simulink model "Smart_City_QCar2_self_driving_stack"  (R2024b)
settings: Solver=ode1  StartTime=0.0  StopTime=inf  FixedStep=Controller_Sample_Time  RelTol=1e-3  EnableMultiTasking=on
values from neighbouring files (symbols this model uses):
  angles_qcar2 = angles_new_qcar2(2: length (angles_new_qcar2), width (angles_new_qcar2)-5)    [Setup_QCar1and2_params.m]
  Audio_Sample_Time = 0.3    [Setup_QCar1and2_params.m]
  cal_pos = [0, 0, 0]    [Setup_QCar1and2_params.m]
  cameraStepSize = 3e-2    (= 0.03)    [Setup_QCar1and2_params.m]
  Cobra_Start = [0 0 0 0 0 0 0 0 0 0 0 0 ... (192000 elements, 192000x1)]    [QCar_Sounds.mat]
  Controller_Sample_Time = CSI_Sample_Time/10    (= 0.00166666666667)    [Setup_QCar1and2_params.m]
  CSI_Sample_Time = 1/60    (= 0.0166666666667)    [Setup_QCar1and2_params.m]
  engine = [0.455749511719 0.619506835938 0.612854003906 0.499603271484 0.347473144531 0.278045654297 0.304656982422 0.258544921875 0.100128173828 0.0902099609375 0.341461181641 0.515716552734 ... (88200 elements, 44100x2)]    [QCar_Sounds.mat]
  GyroKF_P0 = eye(2)    [Setup_QCar1and2_params.m]
  GyroKF_Q = diag([0.01, 0.001])    [Setup_QCar1and2_params.m]
  GyroKF_R = 0.01    [Setup_QCar1and2_params.m]
  GyroKF_X0 = [0;0]    [Setup_QCar1and2_params.m]
  honk = [0.01708984375 0.0179443359375 0.018798828125 0.019775390625 0.0209655761719 0.0218505859375 0.0221557617188 0.0223693847656 0.022705078125 0.023681640625 0.0252075195312 0.0257263183594 ... (43568 elements, 21784x2)]    [QCar_Sounds.mat]
  ImageDisplay_Sample_Time = CSI_Sample_Time*6    (= 0.1)    [Setup_QCar1and2_params.m]
  Initialization_Time = 5    [Setup_QCar1and2_params.m]
  LiDAR_Sample_Time = CSI_Sample_Time*3    (= 0.05)    [Setup_QCar1and2_params.m]
  map_mask = [1 1 1 0 0 1 0]    [Setup_QCar1and2_params.m]
  NN_Sample_Time = RealSense_Sample_Time*1    (= 0.0333333333333)    [Setup_QCar1and2_params.m]
  path_x = [0.826 0.836 0.846 0.856 0.866 0.876 0.886 0.896 0.906 0.916 0.926 0.936 ... (740 elements, 740x1)]    [SDCS_Paths_7.mat]
  path_x2 = [-0.614 -0.604 -0.594 -0.584 -0.574 -0.564 -0.554 -0.544 -0.534 -0.524 -0.514 -0.504 ... (1090 elements, 1090x1)]    [SDCS_Paths_7.mat]
  path_x3 = [-0.614 -0.603821428571 -0.593642857143 -0.583464285714 -0.573285714286 -0.563107142857 -0.552928571429 -0.54275 -0.532571428571 -0.522392857143 -0.512214285714 -0.502035714286 ... (714 elements, 714x1)]    [SDCS_Paths_7.mat]
  path_x4 = [-0.614 -0.604 -0.594 -0.584 -0.574 -0.564 -0.554 -0.544 -0.534 -0.524 -0.514 -0.504 ... (1761 elements, 1761x1)]    [SDCS_Paths_7.mat]
  path_x5 = [1.436 1.42588571429 1.41577142857 1.40565714286 1.39554285714 1.38542857143 1.37531428571 1.3652 1.35508571429 1.34497142857 1.33485714286 1.32474285714 ... (574 elements, 574x1)]    [SDCS_Paths_7.mat]
  path_x6 = [1.436 1.42588571429 1.41577142857 1.40565714286 1.39554285714 1.38542857143 1.37531428571 1.3652 1.35508571429 1.34497142857 1.33485714286 1.32474285714 ... (1288 elements, 1288x1)]    [SDCS_Paths_7.mat]
  path_x7 = [-1.5778487585 -1.56959877056 -1.56127865467 -1.55288878259 -1.54442952915 -1.53590127231 -1.52730439309 -1.51863927561 -1.50990630701 -1.50110587746 -1.49223838016 -1.4833042113 ... (2260 elements, 2260x1)]    [SDCS_Paths_7.mat]
  path_y = [-1.0887 -1.0887 -1.0887 -1.0887 -1.0887 -1.0887 -1.0887 -1.0887 -1.0887 -1.0887 -1.0887 -1.0887 ... (740 elements, 740x1)]    [SDCS_Paths_7.mat]
  path_y2 = [-1.0887 -1.0887 -1.0887 -1.0887 -1.0887 -1.0887 -1.0887 -1.0887 -1.0887 -1.0887 -1.0887 -1.0887 ... (1090 elements, 1090x1)]    [SDCS_Paths_7.mat]
  path_y3 = [-1.0887 -1.0887 -1.0887 -1.0887 -1.0887 -1.0887 -1.0887 -1.0887 -1.0887 -1.0887 -1.0887 -1.0887 ... (714 elements, 714x1)]    [SDCS_Paths_7.mat]
  path_y4 = [-1.0887 -1.0887 -1.0887 -1.0887 -1.0887 -1.0887 -1.0887 -1.0887 -1.0887 -1.0887 -1.0887 -1.0887 ... (1761 elements, 1761x1)]    [SDCS_Paths_7.mat]
  path_y5 = [-0.8157 -0.8157 -0.8157 -0.8157 -0.8157 -0.8157 -0.8157 -0.8157 -0.8157 -0.8157 -0.8157 -0.8157 ... (574 elements, 574x1)]    [SDCS_Paths_7.mat]
  path_y6 = [-0.8157 -0.8157 -0.8157 -0.8157 -0.8157 -0.8157 -0.8157 -0.8157 -0.8157 -0.8157 -0.8157 -0.8157 ... (1288 elements, 1288x1)]    [SDCS_Paths_7.mat]
  path_y7 = [-0.614490295955 -0.61974988896 -0.624981792226 -0.630185771997 -0.635361595765 -0.640509032279 -0.645627851559 -0.6507178249 -0.655778724888 -0.660810325409 -0.665812401655 -0.670784730139 ... (2260 elements, 2260x1)]    [SDCS_Paths_7.mat]
  put_me_down = [0 0 0 0 0 0 0 0 0 0 0 0 ... (335870 elements, 167935x2)]    [QCar_Sounds.mat]
  qcar2_lidar_to_map_rotation = 0    [Setup_QCar1and2_params.m]
  QCarEKF_L = 0.24    [Setup_QCar1and2_params.m]
  QCarEKF_P0 = eye(3)    [Setup_QCar1and2_params.m]
  QCarEKF_Q = diag([0.00001, 0.00001, 0.00001])    [Setup_QCar1and2_params.m]
  QCarEKF_R_combined = diag([0.1, 0.1, 0.01])    [Setup_QCar1and2_params.m]
  QCarEKF_R_heading = diag(0.1)    [Setup_QCar1and2_params.m]
  QcarKF_X0 = [0; 0; 0]    [Setup_QCar1and2_params.m]
  range_qcar2 = distance_new_qcar2(2: length (distance_new_qcar2), width (distance_new_qcar2)-5)    [Setup_QCar1and2_params.m]
  RealSense_Sample_Time = CSI_Sample_Time*2    (= 0.0333333333333)    [Setup_QCar1and2_params.m]
  truck_start = [0.00137329101562 0.00115966796875 0.0006103515625 0.000762939453125 0.00115966796875 0.00198364257812 0.00115966796875 0.000762939453125 0.00137329101562 0.00115966796875 0.00115966796875 0.000762939453125 ... (60000 elements, 60000x1)]    [QCar_Sounds.mat]
undefined symbols (not defined in the file or in its folder): DiscIntNeverNeededParam, gcbh, height, HIL, Joystick_Sample_Time, JPEG, left, Point, qc_get_step_size, top, video_display_show, width
libraries: quarc_library x65, simulink_extras x12, simulink x8
(part 1 of 5)
settings Model: SimulationMode=external  ExtModeTrigDuration=10000  Creator=PKaram  LastModifiedBy=user
settings SolverCC: AlgebraicLoopSolver=TrustRegion  PositivePriorityOrder=on  AutoInsertRateTranBlk=on
settings DataIOCC: ReturnWorkspaceOutputs=off
settings DebuggingCC: ParameterPrecisionLossMsg=none  UnconnectedInputMsg=warning  UnconnectedOutputMsg=warning  UnconnectedLineMsg=warning  ArithmeticOperatorsInVariantConditions=warning
settings HardwareCC: ProdBitPerLong=64  ProdLargestAtomicInteger=LongLong  ProdLargestAtomicFloat=Double  ProdLongLongMode=on  ProdHWDeviceType=ARM Compatible->ARM 64-bit (LP64)
settings ModelReferenceCC: EnableRefExpFcnMdlSchedulingChecks=on
settings SFSimCC: SimUseLocalCustomCode=off  CustomCodeUndefinedFunction=UseInterfaceOnly
settings RTWCC: Description=QUARC Linux QCar2 Target Using Toolchain  SystemTargetFile=quarc_linux_qcar2.tlc  TemplateMakefile=quarc_linux_nvidia_tmf  RTWUseLocalCustomCode=off  Toolchain=QUARC linux_qcar2 | gmake (64-bit Windows)  BuildConfiguration=Faster Runs  GPUComputeCapability=3.5  DLArmComputeVersion=19.05
settings CodeAppCC: StateflowObjectComments=on
settings STFCustomTargetCC: TargetLangStandard=C99 (ISO)  ConcurrentExecutionCompliant=on  GRTInterface=on  UseToolchainInfoCompliant=on  SystemTargetFile=quarc_linux_qcar2.tlc
settings GRTTargetCC: ParMdlRefBuildCompliant=off  CompOptLevelCompliant=off  CombineOutputUpdateFcns=off  MatFileLogging=off  CPPClassGenCompliant=off  GRTInterface=on  ExtMode=on  ExtModeMexFile=quarc_comm  ExtModeMexArgs='-w -d /home/nvidia/Documents -uri %u', 'tcpip://192.168.2.11:17001'
settings ConfigComp: CovMetricSettings=dswe

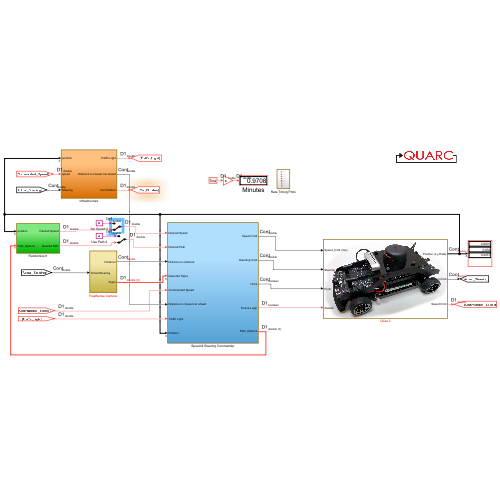
[thumbnail: Simulink's stored preview of the top-level diagram]
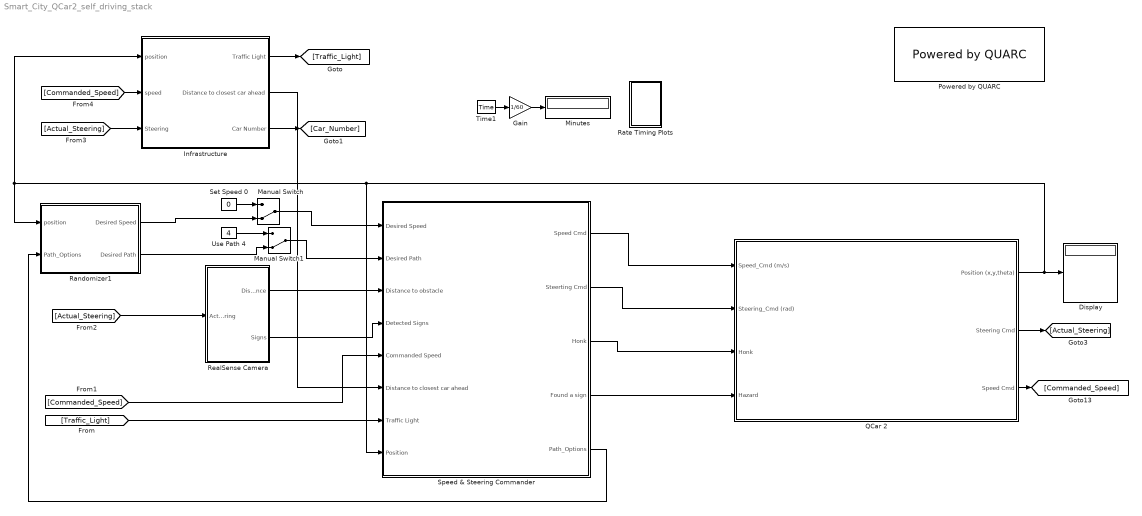
== system Smart_City_QCar2_self_driving_stack ==
  Display : Display
  Gain : Gain  Gain=1/60
  Infrastructure : Subsystem
  Manual Switch : ManualSwitch  CurrentSetting=0
  Manual Switch1 : ManualSwitch  CurrentSetting=0
  Minutes : Display
  Powered by QUARC : quarc_library/Logos/Powered by QUARC
  QCar 2 : Subsystem
      mask Display: image('QCar2.png');
  Randomizer1 : Subsystem
  Rate Timing Plots : Subsystem
  RealSense Camera : Subsystem
  Set Speed 0 : Constant  Value=0
  Speed & Steering Commander : Subsystem
  Time1 : quarc_library/Sources/Time/Time  time_source=Wall clock  sample_time=qc_get_step_size
  Use Path 4 : Constant  Value=4
  wires:
  [Actual_Steering] -> RealSense Camera/1(Actual Steering)
  [Actual_Steering] -> Infrastructure/3(Steering)
  Use Path 4/1 -> Manual Switch1/1
  QCar 2/1(Position (x,y,theta)) -> Randomizer1/1(position), Infrastructure/1(position), Speed & Steering Commander/8(Position), Display/1
  [Traffic_Light] -> Speed & Steering Commander/7(Traffic Light)
  QCar 2/2(Steering Cmd) -> [Actual_Steering]
  Infrastructure/1(Traffic Light) -> [Traffic_Light]
  Randomizer1/1(Desired Speed) -> Manual Switch/2
  [Commanded_Speed] -> Speed & Steering Commander/5(Commanded Speed)
  Time1/1 -> Gain/1
  Manual Switch/1 -> Speed & Steering Commander/1(Desired Speed)
  Manual Switch1/1 -> Speed & Steering Commander/2(Desired Path)
  Speed & Steering Commander/2(Steerting Cmd) -> QCar 2/2(Steering_Cmd (rad))
  Speed & Steering Commander/4(Found a sign) -> QCar 2/4(Hazard)
  Infrastructure/2(Distance to closest car ahead) -> Speed & Steering Commander/6(Distance to closest car ahead)
  Speed & Steering Commander/1(Speed Cmd) -> QCar 2/1(Speed_Cmd (m/s))
  Speed & Steering Commander/5(Path_Options) -> Randomizer1/2(Path_Options)
  Speed & Steering Commander/3(Honk) -> QCar 2/3(Honk)
  Infrastructure/3(Car Number) -> [Car_Number]
  QCar 2/3(Speed Cmd) -> [Commanded_Speed]
  Set Speed 0/1 -> Manual Switch/1
  [Commanded_Speed] -> Infrastructure/2("speed ")
  RealSense Camera/2(Signs) -> Speed & Steering Commander/4(Detected Signs)
  Randomizer1/2(Desired Path) -> Manual Switch1/2
  Gain/1 -> Minutes/1
  RealSense Camera/1(Distance) -> Speed & Steering Commander/3(Distance to obstacle)

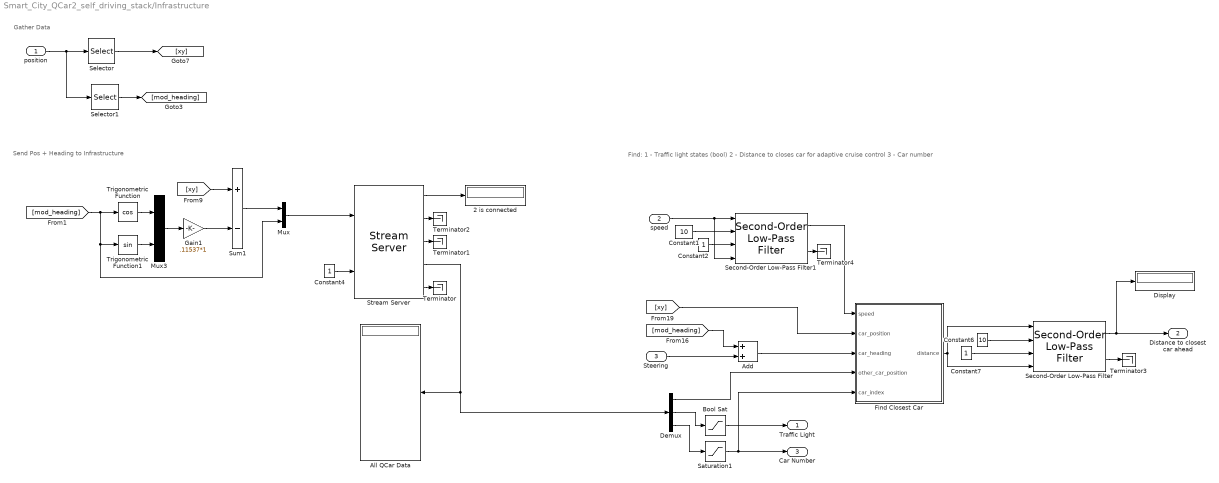
== system Smart_City_QCar2_self_driving_stack/Infrastructure ==
  note: Find:
      | 1 - Traffic light states (bool)
      | 2 - Distance to closes car for adaptive cruise control
      | 3 - Car number
  note: Send Pos + Heading to Infrastructure
  note: Gather Data
  position : Inport
  "speed " : Inport  Port=2
  Steering : Inport  Port=3
  2 is connected : Display
      settings: Decimation=100
  Add : Sum
  All QCar Data : Display
  Bool Sat : Saturate  UpperLimit=1  LowerLimit=0
  Constant1 : Constant  Value=10
  Constant2 : Constant
  Constant4 : Constant
  Constant6 : Constant  Value=10
  Constant7 : Constant
  Demux : Demux  Outputs=[10 1 1]
  Display : Display
  Find Closest Car : Subsystem
  Gain1 : Gain  Gain=.11537*1
  Mux : Mux  Inputs=2
  Mux3 : Mux  Inputs=2
  Saturation1 : Saturate  UpperLimit=5  LowerLimit=1
  Second-Order Low-Pass Filter : quarc_library/Continuous/Second-Order Low-Pass Filter  params_source=External (input ports)  input_width=1  input_zeta=1  input_init=0
  Second-Order Low-Pass Filter1 : quarc_library/Continuous/Second-Order Low-Pass Filter  params_source=External (input ports)  input_width=1  input_zeta=1  input_init=0
  Selector : Selector  InputPortWidth=3  IndexOptions=Index vector (dialog)  Indices=1:2  OutputSizes=1
  Selector1 : Selector  InputPortWidth=3  IndexOptions=Index vector (dialog)  Indices=3  OutputSizes=1
  Stream Server : quarc_library/Communications/Basic/Stream Server  uri_source=Specify via dialog (do not evaluate)  uri=tcpip://remotehost:1111?nagle='off'  send_buffer_size=1460  receive_buffer_size=1460  byte_order=little endian (Intel - LSB first)  optimization=Minimum latency  send_options=Send most recent data  receive_options=Receive most recent data  default_value=10* ones (1,12)  sample_time=qc_get_step_size  active=off  implementation=Use blocking I/O in a separate thread  send_fifo_size=1  receive_fifo_size=1  send_priority=0  receive_priority=0  send_dimensions=off  receive_dimensions=off  max_dimensions=-1  data_type=Inherited via back propagation  type_expr=BusObject
      settings: AttributesFormatString="\"tcpip://remotehost:1111?nagle='off'\""
  Sum1 : Sum  Inputs=+-
  Terminator{,1..4} (5 alike) : Terminator
  Trigonometric Function : Trigonometry  Operator=cos
  Trigonometric Function1 : Trigonometry
  Traffic Light : Outport
  Distance to closest car ahead : Outport  Port=2
  Car Number : Outport  Port=3
  wires:
  Constant7/1 -> Second-Order Low-Pass Filter/3
  Constant4/1 -> Stream Server/2
  Stream Server/1 -> 2 is connected/1
  Constant6/1 -> Second-Order Low-Pass Filter/2
  position/1 -> Selector1/1, Selector/1
  Selector/1 -> [xy]
  Selector1/1 -> [mod_heading]
  Second-Order Low-Pass Filter/1 -> Display/1, Distance to closest car ahead/1
  Constant1/1 -> Second-Order Low-Pass Filter1/2
  "speed "/1 -> Second-Order Low-Pass Filter1/4, Second-Order Low-Pass Filter1/1
  Stream Server/4 -> Demux/1, All QCar Data/1
  [xy] -> Find Closest Car/2(car_position)
  Constant2/1 -> Second-Order Low-Pass Filter1/3
  Second-Order Low-Pass Filter1/1 -> Find Closest Car/1("speed ")
  Find Closest Car/1(distance) -> Second-Order Low-Pass Filter/1, Second-Order Low-Pass Filter/4
  Add/1 -> Find Closest Car/3(car_heading)
  [mod_heading] -> Add/1
  Steering/1 -> Add/2
  Demux/1 -> Find Closest Car/4(other_car_position)
  Demux/2 -> Bool Sat/1
  Bool Sat/1 -> Traffic Light/1
  Mux/1 -> Stream Server/1
  Sum1/1 -> Mux/1
  Demux/3 -> Saturation1/1
  Saturation1/1 -> Find Closest Car/5(car_index), Car Number/1
  [mod_heading] -> Mux/2, Trigonometric Function1/1, Trigonometric Function/1
  Mux3/1 -> Gain1/1
  Trigonometric Function1/1 -> Mux3/2
  [xy] -> Sum1/1
  Gain1/1 -> Sum1/2
  Trigonometric Function/1 -> Mux3/1
  Stream Server/5 -> Terminator/1
  Stream Server/3 -> Terminator1/1
  Stream Server/2 -> Terminator2/1
  Second-Order Low-Pass Filter/2 -> Terminator3/1
  Second-Order Low-Pass Filter1/2 -> Terminator4/1

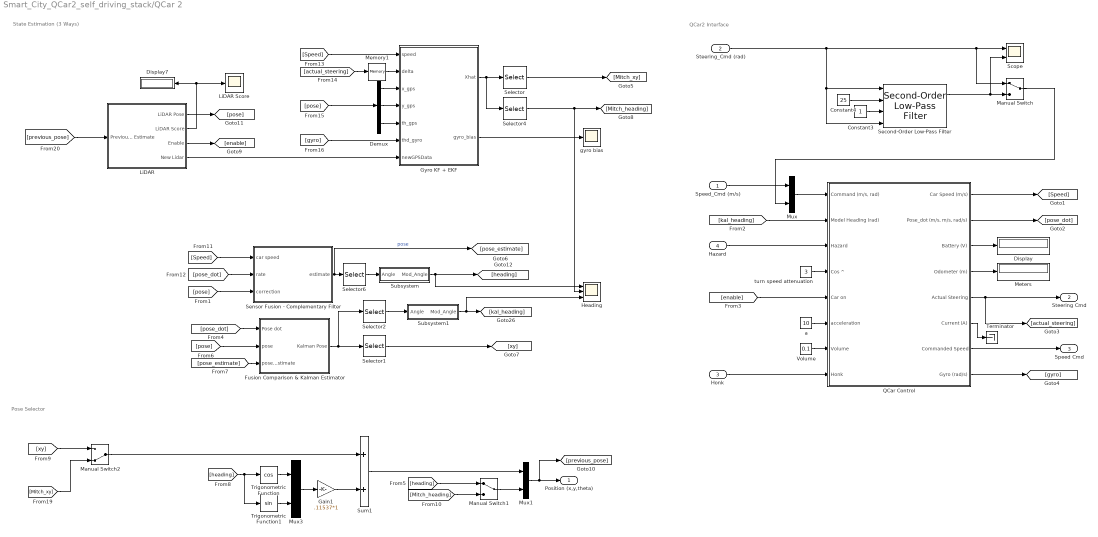
== system Smart_City_QCar2_self_driving_stack/QCar 2 ==
  note: State Estimation (3 Ways)
  note: QCar2 Interface
  note: Pose Selector
  Speed_Cmd (m/s) : Inport
  Steering_Cmd (rad) : Inport  Port=2
  Honk : Inport  Port=3
  Hazard : Inport  Port=4
  Constant3 : Constant
  Constant4 : Constant  Value=25
  Demux : Demux  Outputs=3
  Display : Display
  Display7 : Display
  Fusion Comparison & Kalman Estimator : Subsystem
  Gain1 : Gain  Gain=.11537*1
  Gyro KF + EKF : Subsystem
  Heading : Scope  NumInputPorts=3
  LiDAR : Subsystem
  LiDAR Score : Scope
  Manual Switch : ManualSwitch
  Manual Switch1 : ManualSwitch
  Manual Switch2 : ManualSwitch  CurrentSetting=0
  Memory1 : Memory
  Meters : Display
  Mux : Mux  Inputs=2
  Mux1 : Mux  Inputs=2
  Mux3 : Mux  Inputs=2
  QCar Control : Subsystem
  Scope : Scope  NumInputPorts=2
  Second-Order Low-Pass Filter : quarc_library/Continuous/Second-Order Low-Pass Filter  params_source=External (input ports)  input_width=1  input_zeta=1  input_init=0
  Selector : Selector  InputPortWidth=3  IndexOptions=Index vector (dialog)  Indices=1:2  OutputSizes=1
  Selector1 : Selector  InputPortWidth=3  IndexOptions=Index vector (dialog)  Indices=1:2  OutputSizes=1
  Selector2 : Selector  InputPortWidth=3  IndexOptions=Index vector (dialog)  Indices=3  OutputSizes=1
  Selector4 : Selector  InputPortWidth=3  IndexOptions=Index vector (dialog)  Indices=3  OutputSizes=1
  Selector6 : Selector  InputPortWidth=3  IndexOptions=Index vector (dialog)  Indices=3  OutputSizes=1
  Sensor Fusion - Complementary Filter : Subsystem
  Subsystem : Subsystem
  Subsystem1 : Subsystem
  Sum1 : Sum
  Terminator : Terminator
  Trigonometric Function : Trigonometry  Operator=cos
  Trigonometric Function1 : Trigonometry
  Volume : Constant  Value=0.1
  a : Constant  Value=10
  gyro bias : Scope
  turn speed attenuation : Constant  Value=3
  Position (x,y,theta) : Outport
  Steering Cmd : Outport  Port=2
  Speed Cmd : Outport  Port=3
  wires:
  Mux/1 -> QCar Control/1("Command (m/s, rad)")
  Speed_Cmd (m/s)/1 -> Mux/1
  LiDAR/2("LiDAR Score ") -> LiDAR Score/1, Display7/1
  LiDAR/1(LiDAR Pose) -> [pose]
  LiDAR/3(Enable) -> [enable]
  [pose] -> Fusion Comparison & Kalman Estimator/2(pose)
  [Speed] -> Sensor Fusion - Complementary Filter/1(car speed)
  Sensor Fusion - Complementary Filter/1(estimate) -> [pose_estimate], Selector6/1  "pose"
  [pose_dot] -> Sensor Fusion - Complementary Filter/2(rate)
  Selector6/1 -> Subsystem/1(Angle)
  Fusion Comparison & Kalman Estimator/1(Kalman Pose) -> Selector2/1, Selector1/1
  [pose] -> Sensor Fusion - Complementary Filter/3(correction)
  Subsystem/1(Mod_Angle) -> Heading/1, [heading]
  [pose_estimate] -> Fusion Comparison & Kalman Estimator/3(pose estimate)
  Selector2/1 -> Subsystem1/1(Angle)
  [pose_dot] -> Fusion Comparison & Kalman Estimator/1(Pose dot)
  QCar Control/1(Car Speed (m/s)) -> [Speed]
  QCar Control/2("Pose_dot (m/s, m/s, rad/s)") -> [pose_dot]
  QCar Control/5(Actual Steering) -> [actual_steering], Steering Cmd/1
  QCar Control/7(Commanded Speed) -> Speed Cmd/1
  Selector1/1 -> [xy]
  [kal_heading] -> QCar Control/2(Model Heading (rad))
  Subsystem1/1(Mod_Angle) -> Heading/3, [kal_heading]
  turn speed attenuation/1 -> QCar Control/4(Cos ^)
  a/1 -> QCar Control/6(acceleration)
  [enable] -> QCar Control/5(Car on)
  Volume/1 -> QCar Control/7(Volume)
  Honk/1 -> QCar Control/8(Honk)
  Mux1/1 -> [previous_pose], Position (x,y,theta)/1
  QCar Control/4(Odometer (m)) -> Meters/1
  Hazard/1 -> QCar Control/3(Hazard)
  Gain1/1 -> Sum1/2
  Trigonometric Function/1 -> Mux3/1
  Mux3/1 -> Gain1/1
  Trigonometric Function1/1 -> Mux3/2
  [heading] -> Trigonometric Function1/1, Trigonometric Function/1
  Sum1/1 -> Mux1/1
  Manual Switch/1 -> Mux/2
  Second-Order Low-Pass Filter/1 -> Scope/2, Manual Switch/2
  Steering_Cmd (rad)/1 -> Manual Switch/1, Scope/1, Second-Order Low-Pass Filter/1, Second-Order Low-Pass Filter/4
  Constant3/1 -> Second-Order Low-Pass Filter/3
  Constant4/1 -> Second-Order Low-Pass Filter/2
  Manual Switch1/1 -> Mux1/2
  [heading] -> Manual Switch1/1
  [Mitch_heading] -> Manual Switch1/2
  [Speed] -> Gyro KF + EKF/1(speed)
  Demux/1 -> Gyro KF + EKF/3(x_gps)
  Demux/2 -> Gyro KF + EKF/4(y_gps)
  Demux/3 -> Gyro KF + EKF/5(th_gps)
  [pose] -> Demux/1
  QCar Control/8(Gyro (rad/s)) -> [gyro]
  [gyro] -> Gyro KF + EKF/6(thd_gyro)
  LiDAR/4(New Lidar) -> Gyro KF + EKF/7(newGPSData)
  Gyro KF + EKF/1(Xhat) -> Selector4/1, Selector/1
  Selector4/1 -> Heading/2, [Mitch_heading]
  Gyro KF + EKF/2(gyro_bias) -> gyro bias/1
  Selector/1 -> [Mitch_xy]
  Manual Switch2/1 -> Sum1/1
  [xy] -> Manual Switch2/1
  [Mitch_xy] -> Manual Switch2/2
  [actual_steering] -> Memory1/1
  Memory1/1 -> Gyro KF + EKF/2(delta)
  [previous_pose] -> LiDAR/1(Previous Estimate)
  QCar Control/3(Battery (V)) -> Display/1
  QCar Control/6(Current (A)) -> Terminator/1

== system Smart_City_QCar2_self_driving_stack/Randomizer1 ==
  note: Tunable Params
  position : Inport
  Path_Options : Inport  Port=2
  Base Speed : Constant  Value=.35
  Compare To Constant : simulink/Logic and Bit Operations/Compare To Constant  relop=<  const=0  OutDataTypeStr=boolean
  Compare To Constant1 : simulink/Logic and Bit Operations/Compare To Constant  relop=>  const=-0.75  OutDataTypeStr=boolean
  Compare To Constant2 : simulink/Logic and Bit Operations/Compare To Constant  relop=<  const=-0.9  OutDataTypeStr=boolean
  Display : Display
  Display1 : Display
  Logical Operator : Logic  AllPortsSameDT=off  OutDataTypeStr=boolean
  Logical Operator1 : Logic  AllPortsSameDT=off  OutDataTypeStr=boolean
  MATLAB Function : MATLAB Function  TreatAsAtomicUnit=on
  Memory1 : Memory  InitialCondition=2  InheritSampleTime=on  LinearizeMemory=on  LinearizeAsDelay=on
  Memory2 : Memory  InitialCondition=1  InheritSampleTime=on  LinearizeMemory=on  LinearizeAsDelay=on
  Subsystem1 : Subsystem
  Terminator : Terminator
  Time b/w Path Changes : Constant  Value=3
  X : Selector  InputPortWidth=3  IndexOptions=Index vector (dialog)  Indices=[1]  OutputSizes=1
  Y : Selector  InputPortWidth=3  IndexOptions=Index vector (dialog)  Indices=[2]  OutputSizes=1
  multiply : Product  Inputs=**
  select which path set to use : Subsystem  TreatAsAtomicUnit=on
  Desired Speed : Outport
  Desired Path : Outport  Port=2
  wires:
  Memory1/1 -> MATLAB Function/1(Previous_Path)
  Memory2/1 -> MATLAB Function/2(Previous_Speed)
  Time b/w Path Changes/1 -> Subsystem1/1(Random Period)
  Subsystem1/1(RisingEdgeTrigger) -> MATLAB Function/5(randomize)
  Base Speed/1 -> MATLAB Function/4(Speed_Cmd_Base)
  MATLAB Function/2(Desired_Speed) -> Desired Speed/1, Memory2/1, Display1/1
  MATLAB Function/1(Desired_Path) -> Memory1/1, Desired Path/1, Display/1
  MATLAB Function/3(Accel_Limit) -> Terminator/1
  Logical Operator1/1 -> select which path set to use/Trigger
  Logical Operator/1 -> Logical Operator1/1
  position/1 -> X/1, Y/1
  select which path set to use/1(map mask) -> multiply/1
  Compare To Constant2/1 -> Logical Operator1/2
  X/1 -> Compare To Constant1/1, Compare To Constant/1
  Compare To Constant/1 -> Logical Operator/1
  Compare To Constant1/1 -> Logical Operator/2
  Y/1 -> Compare To Constant2/1
  Path_Options/1 -> multiply/2
  multiply/1 -> MATLAB Function/3(Path_Options)

== system Smart_City_QCar2_self_driving_stack/Rate Timing Plots ==
  Audio : Scope
  CSI : Scope
  Control : Scope
  Image Displays : Scope
  Joystick : Scope  Commented=on
  LCD : Scope
  LiDAR : Scope
  NN Rate : Scope
  RealSense : Scope
  monitorTiming : Subsystem
  monitorTiming1 : Subsystem
  monitorTiming2 : Subsystem
  monitorTiming3 : Subsystem
  monitorTiming4 : Subsystem  Commented=on
  monitorTiming5 : Subsystem
  monitorTiming6 : Subsystem
  monitorTiming7 : Subsystem
  monitorTiming8 : Subsystem
  wires:
  monitorTiming/1(Timing (s)) -> CSI/1
  monitorTiming1/1(Timing (s)) -> Control/1
  monitorTiming3/1(Timing (s)) -> Image Displays/1
  monitorTiming4/1(Timing (s)) -> Joystick/1
  monitorTiming2/1(Timing (s)) -> RealSense/1
  monitorTiming5/1(Timing (s)) -> LiDAR/1
  monitorTiming6/1(Timing (s)) -> NN Rate/1
  monitorTiming7/1(Timing (s)) -> LCD/1
  monitorTiming8/1(Timing (s)) -> Audio/1

== system Smart_City_QCar2_self_driving_stack/RealSense Camera ==
  note: Capture Realsense and do Object Detection
  Actual Steering : Inport
  Constant8 : Constant  Value=50
  Constant9 : Constant
  Image Transform : quarc_library/Image Processing/Generic/Image Transform  algorithm=Colorize  color_theme=KRYGCBMW  min_pixel=0  max_pixel=65535  contour_depth=1  focal_length=308  principal_point=[262 334]  radial_coeffs=[-0.3129 0.0907]  tangential_coeffs=[]  extrapolated_pixel=0  interpolation=nearest  row_coords=0  column_coords=0  output_height=480  output_width=640  angle=0  origin=[240 320]  output_origin=[240 320]  output_data_type=uint8
      settings: AttributesFormatString=(%<algorithm>)  SourceProductName=QUARC Targets
  Newer Depth : Subsystem  LoadFcn=set_param(gcbh, 'UserData', gcb);  StartFcn=video_display_show([gcb, '/Video Display'], 'add', gcb);  mask(Video Compressed Display){algorithm=JPEG, quality=50, sample_time=-1, use_hardware=on}
      mask prompts: algorithm "Compression algorithm:"; quality "Compression quality (0-100):"; sample_time "Sample time (seconds):"; use_hardware "Use hardware acceleration for video display"
      mask help: Displays a video stream on the host, using compression to minimize bandwidth.
      mask init:
      | qc_set_display('Video\nCompressed\nDisplay');
      settings: UndoDeleteFcn=set_param(gcbh, 'UserData', gcb);  OpenFcn=video_display_show([gcb, '/Video Display'], 'show', gcb);  PreDeleteFcn=video_display_show([gcb, '/Video Display'], 'delete');
      settings: CopyFcn=|
      | set_param(gcbh, 'UserData', gcb);
      | set_param(gcbh, 'LinkStatus', 'none');
      settings: NameChangeFcn=|
      | video_display_show([get_param(gcbh, 'UserData'), '/Video Display'], 'rename', [gcb, '/Video Display']);
      | video_display_show([gcb, '/Video Display'], 'add', gcb);
      | set_param(gcbh, 'UserData', gcb);
      mask Help: web(qc_get_block_help_path(gcb));
      mask TypeOptions algorithm: Image Compress/algorithm
      mask TypeOptions quality: Image Compress/quality
      mask TypeOptions sample_time: Video Display/sample_time
      mask TypeOptions use_hardware: Video Display/use_hardware
      mask Display:
      | patch([0.98591 0.98591 0.62618 0.59072 0.56147   0.536   0.536  0.5441 0.56912 0.59207 0.60881 0.62276 0.63527 0.64364  0.6485  0.6485 0.64706 0.64499 0.63662 0.62411 0.61232 0.59837 0.58307 0.56147   0.536   0.536  0.5441  0.5747 0.60953 0.63662 0.67001  0.7034 0.72851 0.75425 0.77927 0.80294 0.82454 0.84119 0.85865 0.87395 0.88574 0.89339  0.8969 0.89969 0.89969 0.89267  0.8816 0.87044 0.85649  0.8384 0.81824 0.80294 0.78764 0.77513 0.76676 0.75776 0.76397 0.77513 0.79178 0.80987 0.82796 0.84326 0.86207 0.98528],[0.18689 0.05522 0.05522 0.05171 0.05171    0.05 0.18338 0.18338 0.19148 0.20435 0.22298 0.24863 0.28589 0.33125 0.38138 0.55139 0.59801 0.63761 0.68189 0.72149 0.74939 0.76694 0.77855 0.79367 0.79952 0.92768 0.92768 0.92768 0.92417 0.92066 0.91364  0.9032 0.89384 0.88106 0.86594 0.85073 0.82634 0.80537 0.77855 0.74363 0.70403 0.65858 0.61079 0.59099 0.41513 0.37202 0.31847 0.29048 0.25556 0.23342  0.2102 0.19382 0.18221 0.17285 0.16943 0.16124  0.1589 0.16241 0.16709 0.17168  0.1787 0.18221 0.18689 0.18689],[0.9,0.90,0.91])
      | patch([0.536 0.52601 0.46823 0.44528 0.41603 0.39101 0.35555 0.33116 0.31451 0.29291  0.2804 0.26717 0.25322 0.23999 0.22406 0.20732 0.19337 0.17528 0.15935 0.14396 0.13217 0.11759 0.10922 0.10085 0.09671 0.09392 0.09041 0.08906 0.08906 0.09464  0.0995 0.10778 0.11894 0.13145 0.14675 0.16349 0.17672 0.19409 0.20732 0.22406 0.23999 0.26159 0.27833 0.29849 0.31793 0.33602 0.35411 0.37085 0.39245 0.41603   0.536   0.536 0.53159 0.46409   0.446 0.42026 0.39587 0.37571 0.36113 0.34925 0.34088 0.33809 0.33809 0.34088 0.34583 0.35627 0.36392 0.38129 0.39587 0.41117 0.42719 0.44672  0.4676 0.48353 0.48353 0.52394   0.536],[0.05 0.04829 0.04712 0.04712 0.04829 0.05063 0.05405 0.05873 0.06107 0.06692 0.07043 0.07619 0.08087 0.08672 0.09482 0.10652 0.11696 0.13325  0.1508 0.17168 0.19499 0.22415 0.25439 0.28472 0.31379 0.35456 0.38489 0.41513 0.58055 0.63878 0.68774 0.72149 0.75641 0.78089 0.80537 0.82859 0.84029 0.85658 0.86594 0.87404  0.8834 0.89267 0.90086 0.90788 0.91247 0.91832 0.92066   0.923 0.92651 0.92768 0.92768 0.79952 0.79952 0.79952 0.79718 0.78899 0.77153 0.75056 0.72149 0.68072 0.62249  0.5549 0.41396 0.37085 0.33242 0.28121 0.25205 0.22181 0.20552 0.19499 0.18572 0.18221 0.17753 0.17636 0.17753  0.1787  0.1787],[0.9,0.90,0.91])
      | disp('Video\nCompressed\nDisplay');
  Rate Transition : RateTransition
  Rate Transition2 : RateTransition
  Rate Transition4 : RateTransition
  RealSense Capture : Subsystem
  Second-Order Low-Pass Filter2 : quarc_library/Continuous/Second-Order Low-Pass Filter  params_source=External (input ports)  input_width=1  input_zeta=1  input_init=0
  Terminator : Terminator
  Transfer Fcn : TransferFcn  Numerator=[10]  Denominator=[1 10]
  obstacleDetection Markham March 22 : Subsystem
  to 16Hz4 : RateTransition  OutPortSampleTime=ImageDisplay_Sample_Time
  Distance : Outport
  Signs : Outport  Port=2
  wires:
  Transfer Fcn/1 -> Rate Transition4/1
  Actual Steering/1 -> Transfer Fcn/1
  Constant9/1 -> Second-Order Low-Pass Filter2/3
  obstacleDetection Markham March 22/2(distance (m)) -> Rate Transition2/1
  Rate Transition2/1 -> Second-Order Low-Pass Filter2/4, Second-Order Low-Pass Filter2/1
  obstacleDetection Markham March 22/1(imageDepthForDisplay) -> to 16Hz4/1
  Second-Order Low-Pass Filter2/2 -> Terminator/1
  RealSense Capture/1(New) -> obstacleDetection Markham March 22/Enable
  RealSense Capture/2(Depth Image) -> obstacleDetection Markham March 22/1(imageDepth)
  Rate Transition4/1 -> obstacleDetection Markham March 22/2(steering (rad))
  Constant8/1 -> Second-Order Low-Pass Filter2/2
  Second-Order Low-Pass Filter2/1 -> Distance/1
  RealSense Capture/3(Sign Probabilities) -> Rate Transition/1
  Rate Transition/1 -> Signs/1
  to 16Hz4/1 -> Image Transform/1
  Image Transform/1 -> Newer Depth/1(In1)

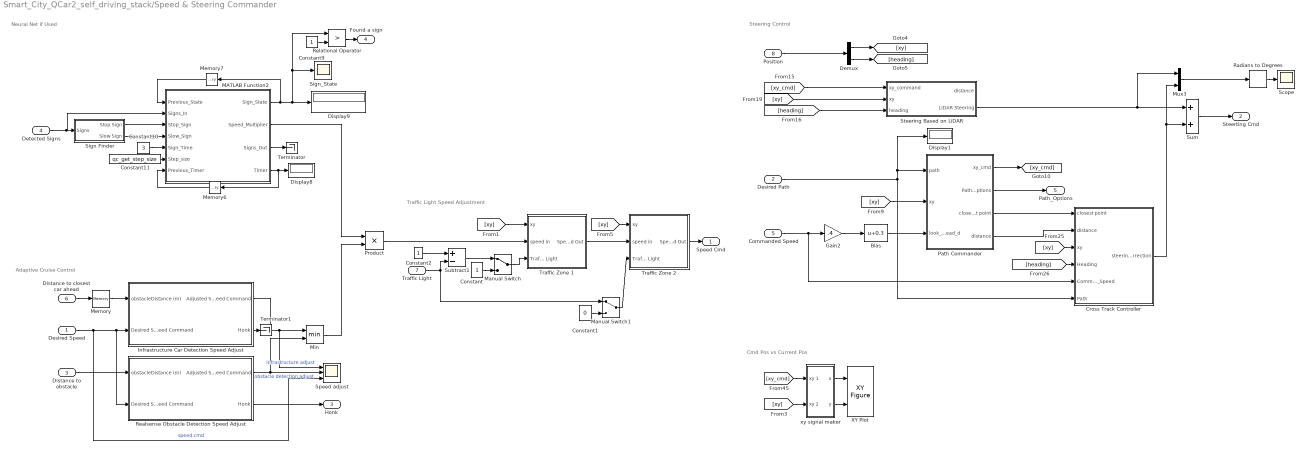
== system Smart_City_QCar2_self_driving_stack/Speed & Steering Commander ==
  note: Steering Control
  note: Cmd Pos vs Current Pos
  note: Traffic Light Speed Adjustment
  note: Neural Net if Used
  note: Adaptive Cruise Control
  Desired Speed : Inport
  Desired Path : Inport  Port=2
  Distance to obstacle : Inport  Port=3
  Detected Signs : Inport  Port=4
  Commanded Speed : Inport  Port=5
  Distance to closest car ahead : Inport  Port=6
  Traffic Light : Inport  Port=7
  Position : Inport  Port=8
  Bias : Bias  Bias=0.3  SaturateOnIntegerOverflow=off
  Constant : Constant
  Constant1 : Constant  Value=0
  Constant10 : Constant  Value=3
  Constant11 : Constant  Value=qc_get_step_size
  Constant2 : Constant
  Constant9 : Constant
  Cross Track Controller : Subsystem
  Demux : Demux  Outputs=2
  Display1 : Display
  Display8 : Display
  Display9 : Display
  Gain2 : Gain  Gain=.4
  Infrastructure Car Detection Speed Adjust : Subsystem
  MATLAB Function2 : MATLAB Function  TreatAsAtomicUnit=on
  Manual Switch : ManualSwitch
  Manual Switch1 : ManualSwitch
  Memory : Memory  InheritSampleTime=on  LinearizeMemory=on  LinearizeAsDelay=on
  Memory6 : Memory  InheritSampleTime=on  LinearizeMemory=on  LinearizeAsDelay=on
  Memory7 : Memory  InitialCondition=1  InheritSampleTime=on  LinearizeMemory=on  LinearizeAsDelay=on
  Min : MinMax  Inputs=2
  Mux3 : Mux  Inputs=2
  Path Commander : Subsystem
  Product : Product
  Radians to Degrees : simulink_extras/Transformations/Radians to Degrees
  Realsense Obstacle Detection Speed Adjust : Subsystem
  Relational Operator : RelationalOperator  Operator=>  OutDataTypeStr=boolean  RndMeth=Simplest  InputSameDT=off
  Scope : Scope
  Sign Finder : Subsystem
  Sign_State : Scope
  Speed adjust : Scope  NumInputPorts=3
  Steering Based on LiDAR : Subsystem
  Subtract1 : Sum  Inputs=+-
  Sum : Sum
  Terminator : Terminator
  Terminator1 : Terminator
  Traffic Zone 1 : Subsystem
  Traffic Zone 2 : Subsystem
  XY Plot : quarc_library/Sinks/Figures/XY Figure  figure_mode=Use figure window  figure_tag=figure1  axes_tag=axes1  plot_mode=Time-based  minimum_x=-2.5  maximum_x=2.5  minimum_y=-2  maximum_y=5  buffer_size=100  update_rate=1  initial_position="1    49  1920   982"  initial_visibility=off  sample_time=-1
      settings: SourceProductName=QUARC Targets
  xy signal maker : Subsystem
  Speed Cmd : Outport
  Steerting Cmd : Outport  Port=2
  Honk : Outport  Port=3
  Found a sign : Outport  Port=4
  Path_Options : Outport  Port=5
  wires:
  [heading] -> Steering Based on LiDAR/3(heading)
  Bias/1 -> Path Commander/3(look_ahead_d)
  Relational Operator/1 -> Found a sign/1
  [xy] -> Cross Track Controller/3(xy)
  Gain2/1 -> Bias/1
  [heading] -> Cross Track Controller/4(Heading)
  Memory6/1 -> MATLAB Function2/7(Previous_Timer)
  Constant9/1 -> Relational Operator/2
  Constant11/1 -> MATLAB Function2/6(Step_size)
  MATLAB Function2/1(Sign_State) -> Display9/1, Relational Operator/1, Sign_State/1, Memory7/1
  Commanded Speed/1 -> Cross Track Controller/5(Commanded_Speed), Gain2/1
  [xy] -> Path Commander/2(xy)
  Mux3/1 -> Radians to Degrees/1
  MATLAB Function2/4(Timer) -> Display8/1, Memory6/1
  Constant10/1 -> MATLAB Function2/5(Sign_Time)
  [xy_cmd] -> Steering Based on LiDAR/1(xy_command)
  Desired Path/1 -> Display1/1, Path Commander/1(path), Cross Track Controller/6(Path)
  Memory7/1 -> MATLAB Function2/1(Previous_State)
  Steering Based on LiDAR/2(LiDAR Steering) -> Mux3/1, Sum/1
  [xy] -> Steering Based on LiDAR/2(xy)
  Path Commander/3(closest point) -> Cross Track Controller/1(closest point)
  Sign Finder/1(Stop Sign) -> MATLAB Function2/3(Stop_Sign)
  Path Commander/1(xy_cmd) -> [xy_cmd]
  Cross Track Controller/1(steering correction) -> Mux3/2, Sum/2
  Radians to Degrees/1 -> Scope/1
  Path Commander/4(distance) -> Cross Track Controller/2(distance)
  Sign Finder/2(Slow Sign) -> MATLAB Function2/4(Slow_Sign)
  Distance to obstacle/1 -> Realsense Obstacle Detection Speed Adjust/1(obstacleDistance (m))
  Desired Speed/1 -> Speed adjust/3, Infrastructure Car Detection Speed Adjust/2(Desired Speed Command), Realsense Obstacle Detection Speed Adjust/2(Desired Speed Command)  "speed cmd"
  Demux/2 -> [heading]
  Position/1 -> Demux/1
  Demux/1 -> [xy]
  Detected Signs/1 -> MATLAB Function2/2(Signs_In), Sign Finder/1(Signs)
  Sum/1 -> Steerting Cmd/1
  MATLAB Function2/2(Speed_Multiplier) -> Product/1
  Realsense Obstacle Detection Speed Adjust/2(Honk) -> Honk/1
  xy signal maker/2(y) -> XY Plot/2
  [xy_cmd] -> xy signal maker/1(xy 1)
  [xy] -> xy signal maker/2(xy 2)
  xy signal maker/1(x) -> XY Plot/1
  Traffic Zone 1/1(Speed Out) -> Traffic Zone 2/2(speed in)
  [xy] -> Traffic Zone 2/1(xy)
  Manual Switch/1 -> Traffic Zone 1/3(Traffic Light)
  [xy] -> Traffic Zone 1/1(xy)
  Traffic Zone 2/1(Speed Out) -> Speed Cmd/1
  Product/1 -> Traffic Zone 1/2(speed in)
  Distance to closest car ahead/1 -> Memory/1
  Min/1 -> Product/2
  Infrastructure Car Detection Speed Adjust/1(Adjusted Speed Command) -> Speed adjust/1, Min/1  "infrastructure adjust"
  Realsense Obstacle Detection Speed Adjust/1(Adjusted Speed Command) -> Min/2, Speed adjust/2  "obstacle detection adjust"
  Memory/1 -> Infrastructure Car Detection Speed Adjust/1(obstacleDistance (m))
  Constant/1 -> Manual Switch/2
  Constant1/1 -> Manual Switch1/2
  Traffic Light/1 -> Manual Switch1/1, Subtract1/2
  Manual Switch1/1 -> Traffic Zone 2/3(Traffic Light)
  Path Commander/2(Path_Options) -> Path_Options/1
  MATLAB Function2/3(Signs_Out) -> Terminator/1
  Infrastructure Car Detection Speed Adjust/2(Honk) -> Terminator1/1
  Constant2/1 -> Subtract1/1
  Subtract1/1 -> Manual Switch/1

== system Smart_City_QCar2_self_driving_stack/Infrastructure/Find Closest Car ==
  "speed " : Inport
  car_position : Inport  Port=2
  car_heading : Inport  Port=3
  other_car_position : Inport  Port=4
  car_index : Inport  Port=5
  Constant1 : Constant  Value=65
  Constant2 : Constant  Value=45
  Constant6 : Constant
  Constant7 : Constant
  Constant8 : Constant  Value=10
  Degrees to Radians : simulink_extras/Transformations/Degrees to Radians
  Demux : Demux  Outputs=2
  Demux1 : Demux  Outputs=2
  Display{,1..3} (4 alike) : Display
      settings: Decimation=100
  MATLAB Function : MATLAB Function  TreatAsAtomicUnit=on
  MATLAB Function1 : MATLAB Function  TreatAsAtomicUnit=on
  Radians to Degrees : simulink_extras/Transformations/Radians to Degrees
  Saturation Dynamic : simulink/Discontinuities/Saturation Dynamic  OutMin=[]  OutMax=[]  OutDataTypeStr=Inherit: Same as second input  OutDataType=fixdt(1, 16)  OutScaling=2^-10  DoSatur=off
  distance : Outport
  wires:
  Constant6/1 -> MATLAB Function/7(proximity_radius)
  Constant8/1 -> MATLAB Function/9(max_distance)
  car_index/1 -> MATLAB Function/5(car_index)
  Radians to Degrees/1 -> Display2/1
  car_heading/1 -> MATLAB Function/6(heading)
  MATLAB Function/2(distance_vector) -> Display1/1
  Degrees to Radians/1 -> MATLAB Function/8(proximity_scan_window)
  MATLAB Function/3(heading_vector) -> Radians to Degrees/1
  MATLAB Function/1(distance) -> Display/1, distance/1
  Demux/1 -> MATLAB Function/1(x_car)
  Demux/2 -> MATLAB Function/2(y_car)
  car_position/1 -> Demux/1
  other_car_position/1 -> Demux1/1
  Demux1/1 -> MATLAB Function/3(x_vector)
  Demux1/2 -> MATLAB Function/4(y_vector)
  "speed "/1 -> MATLAB Function1/1(speed)
  Constant7/1 -> MATLAB Function1/2(max_speed)
  Constant1/1 -> Saturation Dynamic/1, MATLAB Function1/4(max_window)
  Constant2/1 -> Saturation Dynamic/3, MATLAB Function1/3(min_window)
  MATLAB Function1/1(proximity_scan_window) -> Saturation Dynamic/2
  Saturation Dynamic/1 -> Display3/1, Degrees to Radians/1

== system Smart_City_QCar2_self_driving_stack/QCar 2/Fusion Comparison & Kalman Estimator ==
  Pose dot : Inport
  pose : Inport  Port=2
  pose estimate : Inport  Port=3
  Angle mod1 : Subsystem
  Constant : Constant  Value=3
  Data Type Conversion1 : DataTypeConversion  OutDataTypeStr=int32  RndMeth=Round  SaturateOnIntegerOverflow=off
  Data Type Conversion2 : DataTypeConversion  OutDataTypeStr=int32  RndMeth=Round  SaturateOnIntegerOverflow=off
  Heading : Scope
  Integrator : Integrator  ExternalReset=level  InitialConditionSource=external  WrappedStateUpperValue=[20 20 pi]  WrappedStateLowerValue=-[20 20 pi]
  Kalman : Selector  InputPortWidth=3  IndexOptions=Index vector (port)  Indices=[1 3]  OutputSizes=1
  LiDAR : Selector  InputPortWidth=3  IndexOptions=Index vector (port)  Indices=[1 3]  OutputSizes=1
  LiDAR1 : Selector  InputPortWidth=3  IndexOptions=Index vector (port)  Indices=[1 3]  OutputSizes=1
  Memory2 : Memory  InheritSampleTime=on  LinearizeMemory=on  LinearizeAsDelay=on
  Mux : Mux  Inputs=2
  Mux1 : Mux  Inputs=2
  Mux2 : Mux  Inputs=2
  Mux4 : Mux  Inputs=3
  RT : RateTransition  OutPortSampleTime=qc_get_step_size
  RT1 : RateTransition  OutPortSampleTime=qc_get_step_size
  RT2 : RateTransition  OutPortSampleTime=qc_get_step_size
  Radians to Degrees : simulink_extras/Transformations/Radians to Degrees
  Radians to Degrees2 : simulink_extras/Transformations/Radians to Degrees
  Radians to Degrees3 : simulink_extras/Transformations/Radians to Degrees
  Relational Operator1 : RelationalOperator  Operator=~=  OutDataTypeStr=boolean  RndMeth=Simplest  InputSameDT=off
  Scope : Scope  NumInputPorts=3
  Selector1 : Selector  InputPortWidth=3  IndexOptions=Index vector (dialog)  Indices=1:2  OutputSizes=1
  Selector2 : Selector  InputPortWidth=3  IndexOptions=Index vector (dialog)  Indices=3  OutputSizes=1
  Selector3 : Selector  InputPortWidth=3  IndexOptions=Index vector (dialog)  Indices=1:2  OutputSizes=1
  Selector4 : Selector  InputPortWidth=3  IndexOptions=Index vector (dialog)  Indices=3  OutputSizes=1
  Selector5 : Selector  InputPortWidth=3  IndexOptions=Index vector (dialog)  Indices=1:2  OutputSizes=1
  Selector6 : Selector  InputPortWidth=3  IndexOptions=Index vector (dialog)  Indices=3  OutputSizes=1
  Selector7 : Selector  InputPortWidth=3  IndexOptions=Index vector (dialog)  Indices=1  OutputSizes=1
  m_to_mm : Gain  Gain=1e3
  m_to_mm1 : Gain  Gain=1e3
  m_to_mm2 : Gain  Gain=1e3
  Kalman Pose : Outport
  wires:
  Mux2/1 -> LiDAR1/1, Scope/3
  Selector6/1 -> Radians to Degrees3/1
  m_to_mm2/1 -> Mux2/1
  Integrator/1 -> Kalman Pose/1, Selector1/1, Selector2/1  "pose"
  Selector1/1 -> m_to_mm/1
  pose estimate/1 -> Selector6/1, Selector5/1
  Selector5/1 -> m_to_mm2/1
  Selector4/1 -> Radians to Degrees2/1
  Radians to Degrees3/1 -> Mux2/2
  Mux/1 -> Scope/1, Kalman/1, Data Type Conversion2/1
  m_to_mm1/1 -> Mux1/1
  Selector2/1 -> Radians to Degrees/1
  Pose dot/1 -> Integrator/1
  m_to_mm/1 -> Mux/1
  Mux1/1 -> Data Type Conversion1/1, RT/1
  Radians to Degrees/1 -> Mux/2
  Selector3/1 -> m_to_mm1/1
  Radians to Degrees2/1 -> Mux1/2
  RT/1 -> LiDAR/1, Scope/2
  pose/1 -> Selector7/1, Selector4/1, Selector3/1, RT2/1
  RT2/1 -> Integrator/3
  RT1/1 -> Memory2/1, Relational Operator1/2
  Memory2/1 -> Relational Operator1/1
  Selector7/1 -> RT1/1
  Relational Operator1/1 -> Integrator/2
  Mux4/1 -> Angle mod1/1(Angle)
  LiDAR/1 -> Mux4/2
  Kalman/1 -> Mux4/1
  LiDAR1/1 -> Mux4/3
  Constant/1 -> LiDAR1/2, LiDAR/2, Kalman/2
  Angle mod1/1(Mod_Angle) -> Heading/1

== system Smart_City_QCar2_self_driving_stack/QCar 2/Gyro KF + EKF ==
  speed : Inport
  delta : Inport  Port=2
  x_gps : Inport  Port=3
  y_gps : Inport  Port=4
  th_gps : Inport  Port=5
  thd_gyro : Inport  Port=6
  newGPSData : Inport  Port=7
  Heading Kalman Filter : MATLAB Function  TreatAsAtomicUnit=on
  QCar EKF : MATLAB Function  TreatAsAtomicUnit=on
  Xhat : Outport
  gyro_bias : Outport  Port=2
  wires:
  x_gps/1 -> QCar EKF/3(x_gps)
  y_gps/1 -> QCar EKF/4(y_gps)
  Heading Kalman Filter/1(th_hat) -> QCar EKF/5(th_hat)
  newGPSData/1 -> QCar EKF/6(newGPSData), Heading Kalman Filter/3(newGPSData)
  delta/1 -> QCar EKF/2(delta)
  thd_gyro/1 -> Heading Kalman Filter/1(thd_gyro)
  speed/1 -> QCar EKF/1(speed)
  QCar EKF/1(Xhat) -> Xhat/1
  th_gps/1 -> Heading Kalman Filter/2(th_gps)
  Heading Kalman Filter/2(gyro_bias) -> gyro_bias/1

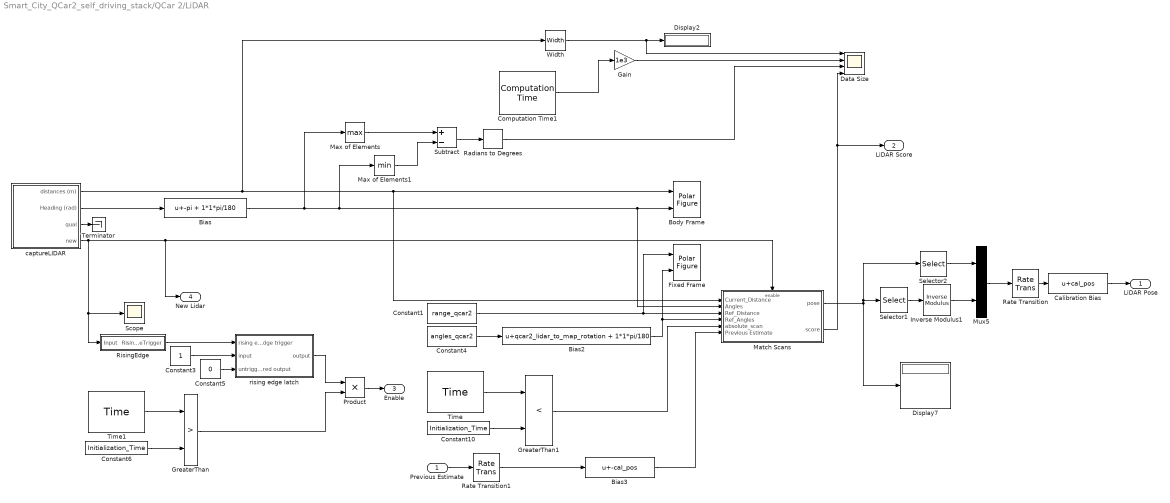
== system Smart_City_QCar2_self_driving_stack/QCar 2/LiDAR ==
  Previous Estimate : Inport
  Bias : Bias  Bias=-pi + 1*1*pi/180  SaturateOnIntegerOverflow=off
  Bias2 : Bias  Bias=qcar2_lidar_to_map_rotation + 1*1*pi/180  SaturateOnIntegerOverflow=off
  Bias3 : Bias  Bias=-cal_pos  SaturateOnIntegerOverflow=off
  Body Frame : quarc_library/Sinks/Figures/Polar Figure  figure_mode=Use figure window  figure_tag=figure1  axes_tag=axes1  plot_mode=Frame-based  minimum_rho=0  maximum_rho=10  minimum_theta=0  maximum_theta=360  zero_location=top  direction=clockwise  buffer_size=SPR_qcar2  update_rate=1  sample_time=-1  initial_position="-958   50  958  973"  initial_visibility=off  line1_style=None  line1_width=0.5  line1_color=[0 0.4470 0.7410]  marker1=Point (.)  marker1_size=1  marker1_edge_color=[0 0.447059 0.741176]  marker1_face_color=[0 0.447059 0.741176]  line2_style=Solid line (-)  line2_width=0.5  line2_color=[0.85098 0.32549 0.0980392]  marker2=None  marker2_size=6  marker2_edge_color=[0.85098 0.32549 0.0980392]  marker2_face_color=[0.85098 0.32549 0.0980392]  line3_style=Solid line (-)  line3_width=0.5  line3_color=[0.929412 0.694118 0.12549]  marker3=None  marker3_size=6  marker3_edge_color=[0.929412 0.694118 0.12549]  marker3_face_color=[0.929412 0.694118 0.12549]  line4_style=Solid line (-)  line4_width=0.5  line4_color=[0.494118 0.184314 0.556863]  marker4=None  marker4_size=6  marker4_edge_color=[0.494118 0.184314 0.556863]  marker4_face_color=[0.494118 0.184314 0.556863]  line5_style=Solid line (-)  line5_width=0.5  line5_color=[0.466667 0.67451 0.188235]  marker5=None  marker5_size=6  marker5_edge_color=[0.466667 0.67451 0.188235]  marker5_face_color=[0.466667 0.67451 0.188235]
      settings: SourceProductName=QUARC Targets
  Calibration Bias : Bias  Bias=cal_pos  SaturateOnIntegerOverflow=off
  Computation Time1 : quarc_library/Sources/Time/Computation Time  sample_time=LiDAR_Sample_Time  use_model=on  use_cpu_time=off
  Constant1 : Constant  Value=range_qcar2
  Constant10 : Constant  Value=Initialization_Time
  Constant3 : Constant
  Constant4 : Constant  Value=angles_qcar2
  Constant5 : Constant  Value=0
  Constant6 : Constant  Value=Initialization_Time
  Data Size : Scope  NumInputPorts=4
  Display2 : Display
  Display7 : Display
  Fixed Frame : quarc_library/Sinks/Figures/Polar Figure  figure_mode=Use figure window  figure_tag=figure1  axes_tag=axes1  plot_mode=Frame-based  minimum_rho=0  maximum_rho=6  minimum_theta=0  maximum_theta=360  zero_location=top  direction=clockwise  buffer_size=SPR_qcar2  update_rate=1  sample_time=-1  initial_position="-1918    50   958   973"  initial_visibility=off  line1_style=None  line1_width=0.5  line1_color=[0 0.4470 0.7410]  marker1=Point (.)  marker1_size=1  marker1_edge_color=[0 0.447059 0.741176]  marker1_face_color=[0 0.447059 0.741176]  line2_style=Solid line (-)  line2_width=0.5  line2_color=[0.85098 0.32549 0.0980392]  marker2=None  marker2_size=6  marker2_edge_color=[0.85098 0.32549 0.0980392]  marker2_face_color=[0.85098 0.32549 0.0980392]  line3_style=Solid line (-)  line3_width=0.5  line3_color=[0.929412 0.694118 0.12549]  marker3=None  marker3_size=6  marker3_edge_color=[0.929412 0.694118 0.12549]  marker3_face_color=[0.929412 0.694118 0.12549]  line4_style=Solid line (-)  line4_width=0.5  line4_color=[0.494118 0.184314 0.556863]  marker4=None  marker4_size=6  marker4_edge_color=[0.494118 0.184314 0.556863]  marker4_face_color=[0.494118 0.184314 0.556863]  line5_style=Solid line (-)  line5_width=0.5  line5_color=[0.466667 0.67451 0.188235]  marker5=None  marker5_size=6  marker5_edge_color=[0.466667 0.67451 0.188235]  marker5_face_color=[0.466667 0.67451 0.188235]
      settings: SourceProductName=QUARC Targets
  Gain : Gain  Gain=1e3
  GreaterThan : RelationalOperator  Operator=>  OutDataTypeStr=boolean  RndMeth=Simplest  InputSameDT=off
  GreaterThan1 : RelationalOperator  Operator=<  OutDataTypeStr=boolean  RndMeth=Simplest  InputSameDT=off
  Inverse Modulus1 : quarc_library/Discontinuities/Inverse Modulus  modulus=2*pi  output_derivative=off  output_revolutions=off  max_x=Inf  min_x=-Inf
  Match Scans : Subsystem
  Max of Elements : MinMax  Function=max
  Max of Elements1 : MinMax
  Mux5 : Mux  Inputs=2
  Product : Product
  Radians to Degrees : simulink_extras/Transformations/Radians to Degrees
  Rate Transition : RateTransition
  Rate Transition1 : RateTransition
  RisingEdge : Subsystem
  Scope : Scope
  Selector1 : Selector  InputPortWidth=3  IndexOptions=Index vector (dialog)  Indices=3  OutputSizes=1
  Selector2 : Selector  InputPortWidth=3  IndexOptions=Index vector (dialog)  Indices=1:2  OutputSizes=1
  Subtract : Sum  Inputs=+-
  Terminator : Terminator
  Time : quarc_library/Sources/Time/Time  time_source=Wall clock  sample_time=LiDAR_Sample_Time
  Time1 : quarc_library/Sources/Time/Time  time_source=Wall clock  sample_time=qc_get_step_size
  Width : Width
  captureLIDAR : Subsystem
  rising edge latch : Subsystem
  LiDAR Pose : Outport
  "LiDAR Score " : Outport  Port=2
  Enable : Outport  Port=3
  New Lidar : Outport  Port=4
  wires:
  Constant1/1 -> Fixed Frame/1, Match Scans/3(Ref_Distance)
  Width/1 -> Display2/1, Data Size/1
  captureLIDAR/1(distances (m)) -> Width/1, Match Scans/1(Current_Distance), Body Frame/1
  Computation Time1/1 -> Gain/1
  Max of Elements/1 -> Subtract/1
  Gain/1 -> Data Size/2
  Max of Elements1/1 -> Subtract/2
  Match Scans/1(pose) -> Selector2/1, Selector1/1, Display7/1
  Inverse Modulus1/1 -> Mux5/2
  Selector2/1 -> Mux5/1
  Radians to Degrees/1 -> Data Size/3
  Selector1/1 -> Inverse Modulus1/1
  Constant6/1 -> GreaterThan/2
  RisingEdge/1(RisingEdgeTrigger) -> rising edge latch/1(rising edge trigger)
  Match Scans/2(score) -> "LiDAR Score "/1, Data Size/4
  Product/1 -> Enable/1
  Constant3/1 -> rising edge latch/2(input)
  Constant5/1 -> rising edge latch/3(untriggered output)
  Constant10/1 -> GreaterThan1/2
  GreaterThan/1 -> Product/2
  Subtract/1 -> Radians to Degrees/1
  Time/1 -> GreaterThan1/1
  GreaterThan1/1 -> Match Scans/5(absolute_scan)
  Time1/1 -> GreaterThan/1
  captureLIDAR/2(Heading (rad)) -> Bias/1
  rising edge latch/1(output) -> Product/1
  Bias/1 -> Max of Elements/1, Max of Elements1/1, Body Frame/2, Match Scans/2(Angles)
  captureLIDAR/4(new) -> RisingEdge/1(Input), Scope/1, Match Scans/Enable, New Lidar/1
  Constant4/1 -> Bias2/1
  Bias2/1 -> Fixed Frame/2, Match Scans/4(Ref_Angles)
  Calibration Bias/1 -> LiDAR Pose/1
  Rate Transition/1 -> Calibration Bias/1
  Mux5/1 -> Rate Transition/1
  Rate Transition1/1 -> Bias3/1
  Bias3/1 -> Match Scans/6(Previous Estimate)
  Previous Estimate/1 -> Rate Transition1/1
  captureLIDAR/3(qual) -> Terminator/1

== system Smart_City_QCar2_self_driving_stack/QCar 2/QCar Control ==
  "Command (m/s, rad)" : Inport
  Model Heading (rad) : Inport  Port=2
  Hazard : Inport  Port=3
  Cos ^ : Inport  Port=4
  Car on : Inport  Port=5
  acceleration : Inport  Port=6
  Volume : Inport  Port=7
  Honk : Inport  Port=8
  Command : Saturate  UpperLimit=[3 .6]  LowerLimit=-[3 .6]
  Constant5 : Constant  Value=-inf
  Constant6 : Constant
  Data Type Conversion : DataTypeConversion  SaturateOnIntegerOverflow=off  RndMeth=Floor
  Demux : Demux  Outputs=2
  Demux1 : Demux  Outputs=2
  Display : Display
      settings: Decimation=100
  Display1 : Display
      settings: Decimation=100
  Memory : Memory
  Mux : Mux  Inputs=2
  Mux1 : Mux  Inputs=2
  Product : Product
  QCar I/O : Subsystem
  Rate Limiter Dynamic : simulink/Discontinuities/Rate Limiter Dynamic
  bicycleModel : Subsystem
  powerConsumptionMonitor : Subsystem
  speedController : Subsystem
  turnSpeedHandling : Subsystem
  Car Speed (m/s) : Outport
  "Pose_dot (m/s, m/s, rad/s)" : Outport  Port=2
  Battery (V) : Outport  Port=3
  Odometer (m) : Outport  Port=4
  Actual Steering : Outport  Port=5
  Current (A) : Outport  Port=6
  Commanded Speed : Outport  Port=7
  Gyro (rad/s) : Outport  Port=8
  wires:
  QCar I/O/2(batteryVoltage (V) [1]) -> Battery (V)/1, powerConsumptionMonitor/2(batteryVoltage (V) [1])
  powerConsumptionMonitor/1(motorPowerConsumption (W) [1]) -> Display/1
  QCar I/O/1(motorCurrent (A) [1]) -> Current (A)/1, powerConsumptionMonitor/1(motorCurrent (A) [1])
  Model Heading (rad)/1 -> bicycleModel/1(heading (rad))
  powerConsumptionMonitor/2(batteryLevel (%) [1]) -> Display1/1
  QCar I/O/4(gyroscopicRates (rad/s)) -> Gyro (rad/s)/1, bicycleModel/4(gyroscope (rad/s))
  bicycleModel/1("poseRate (m/s, m/s, rad/s)") -> "Pose_dot (m/s, m/s, rad/s)"/1
  Product/1 -> QCar I/O/1("motorCmd (%, rad) [2]"), bicycleModel/2("motorCommands (%, rad)"), Demux/1
  Car on/1 -> QCar I/O/2(Arm), speedController/1(arm (0,1)), Mux/1
  QCar I/O/5(Odometer) -> Odometer (m)/1
  [Speed] -> speedController/3(measuredSpeed (m/s))
  Demux/2 -> Actual Steering/1
  Hazard/1 -> Data Type Conversion/1
  Cos ^/1 -> turnSpeedHandling/2(Cos ^)
  Data Type Conversion/1 -> QCar I/O/3(Hazard)
  speedController/1(throttleCmd (%)) -> Product/2
  Mux/1 -> Product/1
  Constant6/1 -> Mux/2
  Volume/1 -> QCar I/O/4(Volume)
  QCar I/O/3(Speed (m/s)) -> [Speed], bicycleModel/3(carSpeed (m/s)), Car Speed (m/s)/1  "v"
  "Command (m/s, rad)"/1 -> Command/1
  Demux1/1 -> Rate Limiter Dynamic/2
  Rate Limiter Dynamic/1 -> Memory/1, Mux1/1
  Constant5/1 -> Rate Limiter Dynamic/3
  acceleration/1 -> Rate Limiter Dynamic/1
  Demux1/2 -> Mux1/2
  turnSpeedHandling/1(Commands) -> Demux1/1
  Mux1/1 -> speedController/2(desiredSpeed (m/s))
  Command/1 -> turnSpeedHandling/1(Commands in)
  Honk/1 -> QCar I/O/5(Honk)
  Memory/1 -> Commanded Speed/1
